simulink model "Utkarsh_2005574_R_W1_P8"  (R2021a)
settings: Solver=FixedStepAuto  StartTime=0.0  StopTime=20  FixedStep=1  RelTol=1e-3
settings Model: Creator=Viraj  LastModifiedBy=Utkarsh Anand
settings SolverCC: AlgebraicLoopSolver=TrustRegion
settings DataIOCC: ExternalInput=[t, lift_state_req]  LoadExternalInput=on  SaveFormat=Array  SignalLogging=off  DSMLogging=off  ReturnWorkspaceOutputs=off
settings DebuggingCC: SFMachineParentedDataDiag=warning

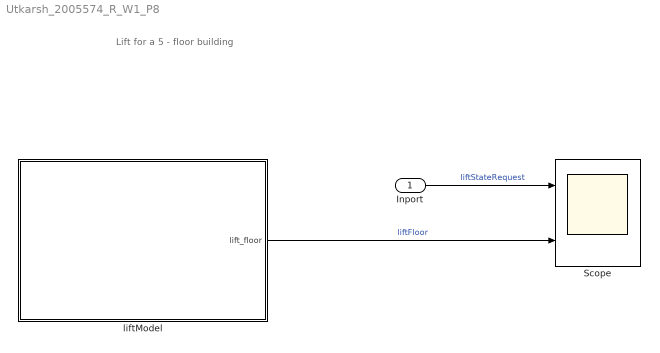
== system Utkarsh_2005574_R_W1_P8 ==
  note: Lift for a 5 - floor building
  Inport : Inport
  Scope : Scope  NumInputPorts=2
  liftModel : Stateflow chart  TreatAsAtomicUnit=on
  wires:
  Inport/1 -> Scope/1  "liftStateRequest"
  liftModel/1(lift_floor) -> Scope/2  "liftFloor"

== stateflow chart Utkarsh_2005574_R_W1_P8/liftModel ==
  state floor = checkFloor [function]
    note: Do not put any code along
        | the transitions that run
        | down the right side!
    (default) -> (junction 111) : % Check Next Floor
    (junction 111) -> (junction 112) [order 1] : [lift_state_req(index) == 0]
    (junction 111) -> (junction 115) [order 2]
    (junction 112) -> (junction 113) : {floor = 0;}
    (junction 113) -> (junction 114)
    (junction 114) -> (junction 118)
    (junction 115) -> (junction 116) [order 1] : [lift_state_req(index) == 1]
    (junction 115) -> (junction 119) [order 2]
    (junction 116) -> (junction 117) : {floor = 1;}
    (junction 117) -> (junction 118)
    (junction 118) -> (junction 122)
    (junction 119) -> (junction 120) [order 1] : [lift_state_req(index) == 2]
    (junction 119) -> (junction 123) [order 2]
    (junction 120) -> (junction 121) : {floor = 2;}
    (junction 121) -> (junction 122)
    (junction 122) -> (junction 126)
    (junction 123) -> (junction 124) [order 1] : [lift_state_req(index) == 3]
    (junction 123) -> (junction 147) [order 2]
    (junction 124) -> (junction 125) : {floor = 3;}
    (junction 125) -> (junction 126)
    (junction 126) -> (junction 128)
    (junction 147) -> (junction 149) [order 1] : [lift_state_req(index) == 4]
    (junction 147) -> (junction 154) [order 2]
    (junction 149) -> (junction 150) : {floor = 4;}
    (junction 150) -> (junction 128)
    (junction 128) -> (junction 157)
    (junction 154) -> (junction 155) [order 1] : [lift_state_req(index) == 5]
    (junction 154) -> (junction 127) [order 2] : {floor = 0}
    (junction 155) -> (junction 156) : {floor = 5;}
    (junction 156) -> (junction 157)
    (junction 157) -> (junction 163)
    (junction 163) -> (junction 127)
    (junction 127) -> (junction 217)
  state running
    state check
      entry:
      lift_floor = checkFloor()
    state ground
    state first
    state second_
    state third_
    state fourth_
    state fifth_
    (default) -> check
    check -> (junction 250)
    (junction 233) -> check : {index = index + 1}
    (junction 250) -> (junction 251)
    (junction 232) -> (junction 233)
    (junction 251) -> ground [order 1] : [lift_floor == 0]
    ground -> (junction 232) : [true]
    (junction 251) -> (junction 249) [order 2]
    (junction 234) -> (junction 232)
    (junction 249) -> first [order 1] : [lift_floor == 1]
    first -> (junction 234) : [true]
    (junction 249) -> (junction 256) [order 2]
    (junction 235) -> (junction 234)
    (junction 256) -> second_ [order 1] : [lift_floor == 2]
    second_ -> (junction 235) : [true]
    (junction 256) -> (junction 255) [order 2]
    (junction 236) -> (junction 235)
    (junction 255) -> third_ [order 1] : [lift_floor == 3]
    third_ -> (junction 236) : [true]
    (junction 255) -> (junction 252) [order 2]
    (junction 237) -> (junction 236)
    (junction 252) -> fourth_ [order 1] : [lift_floor == 4]
    fourth_ -> (junction 237) : [true]
    (junction 252) -> (junction 261) [order 2]
    (junction 240) -> (junction 237)
    (junction 261) -> fifth_ : [lift_floor == 5]
    fifth_ -> (junction 240) : [true]
  state idle
    during:
    if(lift_state_req(index) == -1)
    index = index + 1;
    end
  state end
  state fault
    during:
    lift_floor = 0;
    index = index + 1;
  (default) -> idle
  running -> idle [order 3] : [lift_state_req(index) == -1]
  idle -> running [order 3] : [lift_state_req(index) > -1]
  (junction 25) -> running
  (junction 20) -> (junction 25)
  (junction 18) -> idle : [lift_state_req(index) == -1]
  idle -> (junction 29) [order 2]
  idle -> end [order 1] : [index == 16]
  running -> end [order 1] : [index == 16]
  fault -> end [order 1] : [index ==16]
  running -> (junction 27) [order 2]
  (junction 29) -> fault : [lift_state_req(index) == -2]
  (junction 27) -> fault : [lift_state_req(index) == -2]
  fault -> (junction 18) [order 2]
  fault -> (junction 20) [order 3] : [lift_state_req(index) > -1]
  data: floor function_output; lift_state_req parameter; index local =1; lift_floor output
